simulink model "mnist_softmax_adam_whole_r2017a"  (R2017a)
settings: Solver=FixedStepDiscrete  StartTime=0.0  StopTime=Inf  FixedStep=1  RelTol=1e-3
model workspace (MATLAB code in the model file):
  | BatchSize=100;
  | learningrate=0.05
libraries: ad_blocks x15, simulink x4
settings Model: PauseTimes=2  SnapshotBufferSize=2  SnapshotInterval=1  Creator=percro2  LastModifiedBy=eruffaldi

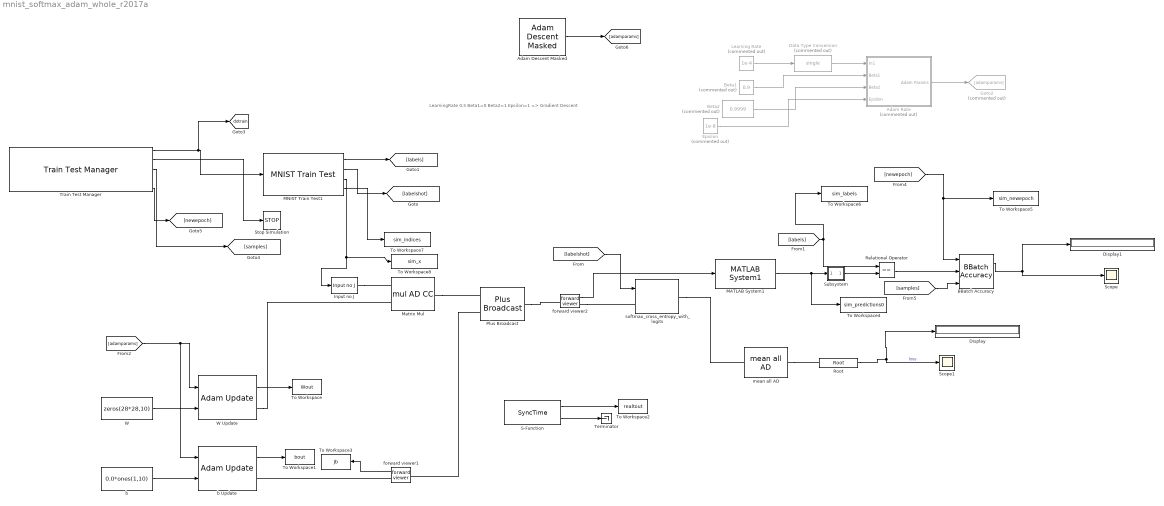
== system mnist_softmax_adam_whole_r2017a ==
  note: LearningRate 0.5 Beta1=0 Beta2=1 Epsilon=1 => Gradient Descent
  Adam Descent Masked : ad_blocks/Adam Descent Masked  learningrate=0.5  beta1=0.9  beta2=0.9999  epsilon=1e-8  adam=off
  Adam Rate : Subsystem  Commented=on
  BBatch Accuracy : ad_blocks/BBatch Accuracy
  Beta1 : Constant  Commented=on  Value=0.9
  Beta2 : Constant  Commented=on  Value=0.9999
  Data Type Conversion : DataTypeConversion  Commented=on  OutDataTypeStr=single
  Display : Display
  Display1 : Display
  Epsilon : Constant  Commented=on  Value=1e-8
  Goto2 : Goto  Commented=on  GotoTag=adamparams
  Input no J : ad_blocks/Input no J  SystemSampleTime=-1
  Learning Rate : Constant  Commented=on  Value=1e-4
  MATLAB System1 : ad_blocks/MATLAB System1  SimulateUsing=Interpreted execution
  MNIST Train Test1 : ad_blocks/MNIST Train Test
  Matrix Mul : ad_blocks/mul AD CC
  Plus Broadcast : ad_blocks/Plus Broadcast
  Relational Operator : RelationalOperator  Operator===  OutDataTypeStr=boolean  RndMeth=Simplest
  Root : ad_blocks/Root  Description=Top level AD block: gets the incoming value, pushes the scalar 1 gradient  SystemSampleTime=-1
  S-Function : S-Function  Priority=1024  FunctionName=SyncTime  Parameters=dt  SFunctionDeploymentMode=off  EnableBusSupport=off  mask{dt=0}
      mask prompts: dt "Period (s) or 0 for sleepless"
      mask Display:
      | port_label('output',1,'Unix Epoch s');
      | port_label('output',2,'Slept s');
  Scope : Scope
  Scope1 : Scope
  Stop Simulation : Stop
  Subsystem : Subsystem
  Terminator : Terminator
  To Workspace : ToWorkspace  VariableName=Wout  SaveFormat=Timeseries  SampleTime=-1
      settings: MaxDataPoints=1
  To Workspace1 : ToWorkspace  VariableName=bout  SaveFormat=Timeseries  SampleTime=-1
      settings: MaxDataPoints=1
  To Workspace2 : ToWorkspace  VariableName=realtout  SaveFormat=Timeseries  SampleTime=1
  To Workspace3 : ToWorkspace  VariableName=Jb  SaveFormat=Timeseries  SampleTime=-1
  To Workspace4 : ToWorkspace  VariableName=sim_predictions0  SaveFormat=Timeseries  SampleTime=-1
  To Workspace5 : ToWorkspace  VariableName=sim_newepoch  SaveFormat=Timeseries  SampleTime=-1
  To Workspace6 : ToWorkspace  VariableName=sim_labels  SaveFormat=Timeseries  SampleTime=-1
  To Workspace7 : ToWorkspace  VariableName=sim_indices  SaveFormat=Timeseries  SampleTime=-1
      settings: MaxDataPoints=1
  To Workspace8 : ToWorkspace  VariableName=sim_x  SaveFormat=Timeseries  SampleTime=-1
      settings: MaxDataPoints=1
  Train Test Manager : ad_blocks/Train Test Manager  testsize=10000  trainsize=60000  skiptrain=0  epochs=2  batchsize=BatchSize  SimulateUsing=Code generation
  W : Constant  Value=zeros(28*28,10)  OutDataTypeStr=single
  W Update : ad_blocks/Adam Update
  b : Constant  Value=0.0*ones(1,10)  OutDataTypeStr=single
  b Update : ad_blocks/Adam Update
  forward viewer1 : ad_blocks/forward viewer  SystemSampleTime=-1
  forward viewer2 : ad_blocks/forward viewer  SystemSampleTime=-1
  mean all AD : ad_blocks/mean all AD
  softmax_cross_entropy_with_logits : ad_blocks/softmax_cross_entropy_with_logits
  tag scope: dotrain=global
  wires:
  Root/1 -> Display/1, Scope1/1  "loss"
  [adamparams] -> b Update/1, W Update/1
  W/1 -> W Update/2
  W Update/1 -> To Workspace/1
  b Update/1 -> To Workspace1/1
  MATLAB System1/1 -> Subsystem/1(In1), To Workspace4/1
  [labelshot] -> softmax_cross_entropy_with_logits/1
  [labels] -> To Workspace6/1, Relational Operator/1
  b/1 -> b Update/2
  S-Function/1 -> To Workspace2/1
  S-Function/2 -> Terminator/1
  Learning Rate/1 -> Data Type Conversion/1
  Adam Rate/1(Adam Params) -> Goto2/1
  forward viewer1/1 -> To Workspace3/1
  Beta1/1 -> Adam Rate/2(Beta1)
  Beta2/1 -> Adam Rate/3(Beta2)
  Epsilon/1 -> Adam Rate/4(Epsilon)
  Data Type Conversion/1 -> Adam Rate/1(In1)
  Train Test Manager/2 -> Stop Simulation/1
  Train Test Manager/1 -> [dotrain], MNIST Train Test1/1
  MNIST Train Test1/3 -> To Workspace8/1, Input no J/1
  Train Test Manager/3 -> [samples]
  MNIST Train Test1/1 -> [labels]
  MNIST Train Test1/2 -> [labelshot]
  Train Test Manager/5 -> [newepoch]
  [newepoch] -> BBatch Accuracy/1, To Workspace5/1
  forward viewer2/1 -> MATLAB System1/1
  MNIST Train Test1/4 -> To Workspace7/1
  BBatch Accuracy/1 -> Display1/1, Scope/1
  Relational Operator/1 -> BBatch Accuracy/2
  [samples] -> BBatch Accuracy/3
  Subsystem/1(Out1) -> Relational Operator/2
  Adam Descent Masked/1 -> [adamparams]
  connections:
  Input no J/RConn1 -- Matrix Mul/LConn1
  W Update/RConn1 -- Matrix Mul/LConn2
  mean all AD/RConn1 -- Root/LConn1
  Matrix Mul/RConn1 -- Plus Broadcast/LConn1
  Plus Broadcast/LConn2 -- forward viewer1/LConn1
  forward viewer1/RConn1 -- b Update/RConn1
  forward viewer2/RConn1 -- softmax_cross_entropy_with_logits/LConn1
  Plus Broadcast/RConn1 -- forward viewer2/LConn1
  softmax_cross_entropy_with_logits/RConn1 -- mean all AD/LConn1

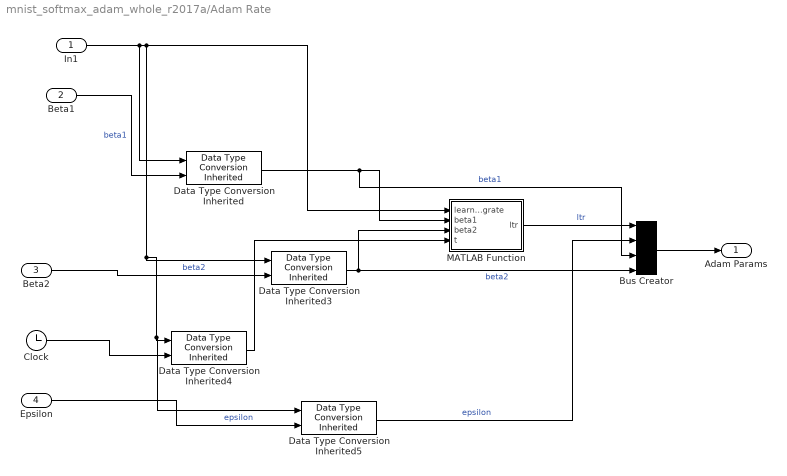
== system mnist_softmax_adam_whole_r2017a/Adam Rate ==
  In1 : Inport
  Beta1 : Inport  Port=2
  Beta2 : Inport  Port=3
  Epsilon : Inport  Port=4
  Bus Creator : BusCreator  Inputs=4
  Clock : Clock
  Data Type Conversion Inherited{,3..5} (4 alike) : simulink/Signal Attributes/Data Type Conversion Inherited  ConvertRealWorld=Real World Value  DoSatur=off
      settings: SourceProductName=Simulink  SourceProductBaseCode=SL
  MATLAB Function : MATLAB Function  TreatAsAtomicUnit=on
  Adam Params : Outport
  wires:
  MATLAB Function/1(ltr) -> Bus Creator/1  "ltr"
  Bus Creator/1 -> Adam Params/1
  Data Type Conversion Inherited/1 -> Bus Creator/3, MATLAB Function/2(beta1)  "beta1"
  In1/1 -> Data Type Conversion Inherited/1, Data Type Conversion Inherited5/1, Data Type Conversion Inherited4/1, Data Type Conversion Inherited3/1, MATLAB Function/1(learningrate)
  Beta1/1 -> Data Type Conversion Inherited/2  "beta1"
  Beta2/1 -> Data Type Conversion Inherited3/2  "beta2"
  Data Type Conversion Inherited3/1 -> MATLAB Function/3(beta2), Bus Creator/4  "beta2"
  Clock/1 -> Data Type Conversion Inherited4/2
  Data Type Conversion Inherited4/1 -> MATLAB Function/4(t)
  Epsilon/1 -> Data Type Conversion Inherited5/2  "epsilon"
  Data Type Conversion Inherited5/1 -> Bus Creator/2  "epsilon"

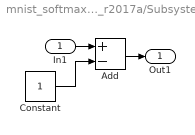
== system mnist_softmax_adam_whole_r2017a/Subsystem ==
  In1 : Inport
  Add : Sum  Inputs=+-
  Constant : Constant  OutDataTypeStr=Inherit: Inherit via back propagation
  Out1 : Outport
  wires:
  In1/1 -> Add/1
  Add/1 -> Out1/1
  Constant/1 -> Add/2

== matlab function mnist_softmax_adam_whole_r2017a/Adam Rate/MATLAB Function ==
  data: learningrate input; ltr output; beta1 input; beta2 input; t input
function ltr = fcn(learningrate,beta1,beta2,t)

if beta1 == 1 || beta2 == 1
    ltr = -learningrate;
else
    ltr = - learningrate * sqrt(1 - beta2^t) / (1 - beta1^t);
end
